simulink model "bh_SM_quad_and_PEND"  (R2019b)
settings: Solver=ode23t  StartTime=0.0  StopTime=200  FixedStep=0.001  RelTol=1e-5  EnableMultiTasking=on
values from neighbouring files (symbols this model uses):
  K = [0.0865712753524 0.00277244570809 -0.0192153083791 -0.00162453351485 3.32348361895e-08 -1.41900444311e-08 -0.0932413563659 2.38058592401e-06 6.56188614095e-09 -0.0932413743514 2.52459639721e-09 9.53911962763e-08 ... (84 elements, 4x21)]    [CONFIRMED_bh_CONT_DES_RESULTS.mat]    (also in CONFIRMED_bh_CONT_DES_RESULTS_DISCRETE.mat = [-4.44584196463e-19 1.60298866655e-18 6.22915677006e-18 0 -9; CONFIRMED_bh_CONT_DES_RESULTS_DISCRETE_PRE_19a_using_DARE_SOLVER.mat = [-0.000193022438438 0.000285510081841 0.000531074046333 0.00; CONFIRMED_bh_CONT_DES_RESULTS_DISCRETE_R2019b.mat = [3.0073494701e-20 1.31173839205e-18 -5.80308139081e-19 0 8.7; CONFIRMED_bh_CONT_DES_RESULTS_PRE_19a_using_CARE_SOLVER.mat = [3.8473936011e-07 5.10337913269e-05 5.50269068807e-05 0.0072)
  xme_dot_0 = (bRg .') * Vm_0(:)    [bh_func_for_lagr_mask_init.m]
undefined symbols (not defined in the file or in its folder): P_elec, P_mot, P_one_prop, P_pend, P_rot, P_veh, P_veh_no_props, sigbuilder_block, X, Y, Z
libraries: fl_lib x85, nesl_utility x39, sm_lib x30, simulink_extras x15, simulink x7, fl_ps_legacy_lib x7, bh_6dof_LIBRARY x1
(part 4 of 4)

== system bh_SM_quad_and_PEND/MODEL_SYS/bh_6DOF (Simscape)/Propellers/MOT_AERO_PROP_1/TQ_on_propeller/DC_mot_elec1 ==
  note: DC Motor - First Principle Equations
  note: L di/dt = V - R i - K_{emf}\fontsize{20}\omega
  PS Constant : fl_lib/Physical Signals/Sources/PS Constant  constant=L
      settings: AttributesFormatString=%<constant>
  PS Divide : fl_ps_legacy_lib/Legacy Physical Signals/Functions/PS Divide
      settings: SourceProductName=Simscape  SourceProductBaseCode=SS  InternalSimscapePortConfiguration="{\"Bottom\":[],\"Left\":[{\"id\":\"I1\",\"label\":\"\",\"type\":\"input\"},{\"id\":\"I2\",\"label\":\"\",\"type\":\"input\"}],\"Right\":[{\"id\":\"O\",\"label\":\"\",\"type\":\"output\"}],\"Top\":[]}"
  PS Gain1 : fl_ps_legacy_lib/Legacy Physical Signals/Functions/PS Gain  gain=Kb
      settings: AttributesFormatString=GAIN= %<gain>  SourceProductName=Simscape
  PS Gain2 : fl_ps_legacy_lib/Legacy Physical Signals/Functions/PS Gain  gain=R
      settings: AttributesFormatString=GAIN= %<gain>  SourceProductName=Simscape
  PS Gain3 : fl_ps_legacy_lib/Legacy Physical Signals/Functions/PS Gain  gain=K
      settings: AttributesFormatString=GAIN= %<gain>  SourceProductName=Simscape
  PS Integrator : fl_ps_legacy_lib/Legacy Physical Signals/Linear Operators/PS Integrator  x0=0
      settings: SourceProductName=Simscape  SourceProductBaseCode=SS  InternalSimscapePortConfiguration="{\"Bottom\":[],\"Left\":[{\"id\":\"I\",\"label\":\"\",\"type\":\"input\"}],\"Right\":[{\"id\":\"O\",\"label\":\"\",\"type\":\"output\"}],\"Top\":[]}"
  PS Subtract1 : fl_ps_legacy_lib/Legacy Physical Signals/Functions/PS Subtract
      settings: SourceProductName=Simscape  SourceProductBaseCode=SS
  PS Subtract2 : fl_ps_legacy_lib/Legacy Physical Signals/Functions/PS Subtract
      settings: SourceProductName=Simscape  SourceProductBaseCode=SS
  V : PMIOPort  Side=Left
  W : PMIOPort  Port=2  Side=Left
  Ki : PMIOPort  Port=3  Side=Right
  connections:
  PS Subtract1/LConn1 -- V/RConn1
  PS Gain1/RConn1 -- PS Subtract1/LConn2
  W/RConn1 -- PS Gain1/LConn1
  PS Subtract2/LConn1 -- PS Subtract1/RConn1
  PS Gain2/RConn1 -- PS Subtract2/LConn2
  PS Integrator/RConn1 -- PS Gain3/LConn1 -- PS Gain2/LConn1
  PS Divide/RConn1 -- PS Integrator/LConn1
  PS Subtract2/RConn1 -- PS Divide/LConn1
  PS Constant/RConn1 -- PS Divide/LConn2
  Ki/RConn1 -- PS Gain3/RConn1

== system bh_SM_quad_and_PEND/MODEL_SYS/bh_6DOF (Simscape)/Propellers/MOT_AERO_PROP_2/TQ_on_propeller/DC_mot_elec ==
  note: DC Motor - First Principle Equations
  note: L di/dt = V - R i - K_{emf}\fontsize{20}\omega
  PS Constant : fl_lib/Physical Signals/Sources/PS Constant  constant=L H
      settings: AttributesFormatString=|
      | %<constant>
      | UNITS = %<constant_unit>
  PS Divide : fl_lib/Physical Signals/Functions/PS Divide
      settings: SourceProductName=Simscape  SourceProductBaseCode=SS
  PS Gain1 : fl_lib/Physical Signals/Functions/PS Gain  gain=Kb V*s/rad
      settings: AttributesFormatString=|
      | GAIN= %<gain>
      | UNITS = %<gain_unit>
  PS Gain2 : fl_lib/Physical Signals/Functions/PS Gain  gain=R Ohm
      settings: AttributesFormatString=|
      | GAIN= %<gain>
      | UNITS = %<gain_unit>
  PS Gain3 : fl_lib/Physical Signals/Functions/PS Gain  gain=K N*m/A
      settings: AttributesFormatString=|
      | GAIN= %<gain>
      | UNITS = %<gain_unit>
  PS Integrator : fl_lib/Physical Signals/Linear Operators/PS Integrator  x0=0 A
      settings: AttributesFormatString=UNITS = %<x0_unit>  SourceProductName=Simscape  SourceProductBaseCode=SS
  PS Subtract1 : fl_lib/Physical Signals/Functions/PS Subtract
      settings: SourceProductName=Simscape
  PS Subtract2 : fl_lib/Physical Signals/Functions/PS Subtract
      settings: SourceProductName=Simscape
  V : PMIOPort  Side=Left
  W : PMIOPort  Port=2  Side=Left
  Ki : PMIOPort  Port=3  Side=Right
  connections:
  PS Subtract1/LConn1 -- V/RConn1
  PS Gain1/RConn1 -- PS Subtract1/LConn2
  W/RConn1 -- PS Gain1/LConn1
  PS Subtract2/LConn1 -- PS Subtract1/RConn1
  PS Gain2/RConn1 -- PS Subtract2/LConn2
  PS Integrator/RConn1 -- PS Gain3/LConn1 -- PS Gain2/LConn1
  PS Divide/RConn1 -- PS Integrator/LConn1
  PS Subtract2/RConn1 -- PS Divide/LConn1
  PS Constant/RConn1 -- PS Divide/LConn2
  Ki/RConn1 -- PS Gain3/RConn1

== system bh_SM_quad_and_PEND/MODEL_SYS/bh_6DOF (Simscape)/Propellers/MOT_AERO_PROP_2/TQ_on_propeller/DC_mot_elec1 ==
  note: DC Motor - First Principle Equations
  note: L di/dt = V - R i - K_{emf}\fontsize{20}\omega
  PS Constant : fl_lib/Physical Signals/Sources/PS Constant  constant=L
      settings: AttributesFormatString=%<constant>
  PS Divide : fl_lib/Physical Signals/Functions/PS Divide
      settings: SourceProductName=Simscape  SourceProductBaseCode=SS
  PS Gain1 : fl_lib/Physical Signals/Functions/PS Gain  gain=Kb
      settings: AttributesFormatString=GAIN= %<gain>
  PS Gain2 : fl_lib/Physical Signals/Functions/PS Gain  gain=R
      settings: AttributesFormatString=GAIN= %<gain>
  PS Gain3 : fl_lib/Physical Signals/Functions/PS Gain  gain=K
      settings: AttributesFormatString=GAIN= %<gain>
  PS Integrator : fl_lib/Physical Signals/Linear Operators/PS Integrator  x0=0 s
      settings: SourceProductName=Simscape  SourceProductBaseCode=SS
  PS Subtract1 : fl_lib/Physical Signals/Functions/PS Subtract
      settings: SourceProductName=Simscape
  PS Subtract2 : fl_lib/Physical Signals/Functions/PS Subtract
      settings: SourceProductName=Simscape
  V : PMIOPort  Side=Left
  W : PMIOPort  Port=2  Side=Left
  Ki : PMIOPort  Port=3  Side=Right
  connections:
  PS Subtract1/LConn1 -- V/RConn1
  PS Gain1/RConn1 -- PS Subtract1/LConn2
  W/RConn1 -- PS Gain1/LConn1
  PS Subtract2/LConn1 -- PS Subtract1/RConn1
  PS Gain2/RConn1 -- PS Subtract2/LConn2
  PS Integrator/RConn1 -- PS Gain3/LConn1 -- PS Gain2/LConn1
  PS Divide/RConn1 -- PS Integrator/LConn1
  PS Subtract2/RConn1 -- PS Divide/LConn1
  PS Constant/RConn1 -- PS Divide/LConn2
  Ki/RConn1 -- PS Gain3/RConn1

== system bh_SM_quad_and_PEND/MODEL_SYS/bh_6DOF (Simscape)/Propellers/MOT_AERO_PROP_3/TQ_on_propeller/DC_mot_elec ==
  note: DC Motor - First Principle Equations
  note: L di/dt = V - R i - K_{emf}\fontsize{20}\omega
  PS Constant : fl_lib/Physical Signals/Sources/PS Constant  constant=L H
      settings: AttributesFormatString=|
      | %<constant>
      | UNITS = %<constant_unit>
  PS Divide : fl_lib/Physical Signals/Functions/PS Divide
      settings: SourceProductName=Simscape  SourceProductBaseCode=SS
  PS Gain1 : fl_lib/Physical Signals/Functions/PS Gain  gain=Kb V*s/rad
      settings: AttributesFormatString=|
      | GAIN= %<gain>
      | UNITS = %<gain_unit>
  PS Gain2 : fl_lib/Physical Signals/Functions/PS Gain  gain=R Ohm
      settings: AttributesFormatString=|
      | GAIN= %<gain>
      | UNITS = %<gain_unit>
  PS Gain3 : fl_lib/Physical Signals/Functions/PS Gain  gain=K N*m/A
      settings: AttributesFormatString=|
      | GAIN= %<gain>
      | UNITS = %<gain_unit>
  PS Integrator : fl_lib/Physical Signals/Linear Operators/PS Integrator  x0=0 A
      settings: AttributesFormatString=UNITS = %<x0_unit>  SourceProductName=Simscape  SourceProductBaseCode=SS
  PS Subtract1 : fl_lib/Physical Signals/Functions/PS Subtract
      settings: SourceProductName=Simscape
  PS Subtract2 : fl_lib/Physical Signals/Functions/PS Subtract
      settings: SourceProductName=Simscape
  V : PMIOPort  Side=Left
  W : PMIOPort  Port=2  Side=Left
  Ki : PMIOPort  Port=3  Side=Right
  connections:
  PS Subtract1/LConn1 -- V/RConn1
  PS Gain1/RConn1 -- PS Subtract1/LConn2
  W/RConn1 -- PS Gain1/LConn1
  PS Subtract2/LConn1 -- PS Subtract1/RConn1
  PS Gain2/RConn1 -- PS Subtract2/LConn2
  PS Integrator/RConn1 -- PS Gain3/LConn1 -- PS Gain2/LConn1
  PS Divide/RConn1 -- PS Integrator/LConn1
  PS Subtract2/RConn1 -- PS Divide/LConn1
  PS Constant/RConn1 -- PS Divide/LConn2
  Ki/RConn1 -- PS Gain3/RConn1

== system bh_SM_quad_and_PEND/MODEL_SYS/bh_6DOF (Simscape)/Propellers/MOT_AERO_PROP_3/TQ_on_propeller/DC_mot_elec1 ==
  note: DC Motor - First Principle Equations
  note: L di/dt = V - R i - K_{emf}\fontsize{20}\omega
  PS Constant : fl_lib/Physical Signals/Sources/PS Constant  constant=L
      settings: AttributesFormatString=%<constant>
  PS Divide : fl_lib/Physical Signals/Functions/PS Divide
      settings: SourceProductName=Simscape  SourceProductBaseCode=SS
  PS Gain1 : fl_lib/Physical Signals/Functions/PS Gain  gain=Kb
      settings: AttributesFormatString=GAIN= %<gain>
  PS Gain2 : fl_lib/Physical Signals/Functions/PS Gain  gain=R
      settings: AttributesFormatString=GAIN= %<gain>
  PS Gain3 : fl_lib/Physical Signals/Functions/PS Gain  gain=K
      settings: AttributesFormatString=GAIN= %<gain>
  PS Integrator : fl_lib/Physical Signals/Linear Operators/PS Integrator  x0=0 s
      settings: SourceProductName=Simscape  SourceProductBaseCode=SS
  PS Subtract1 : fl_lib/Physical Signals/Functions/PS Subtract
      settings: SourceProductName=Simscape
  PS Subtract2 : fl_lib/Physical Signals/Functions/PS Subtract
      settings: SourceProductName=Simscape
  V : PMIOPort  Side=Left
  W : PMIOPort  Port=2  Side=Left
  Ki : PMIOPort  Port=3  Side=Right
  connections:
  PS Subtract1/LConn1 -- V/RConn1
  PS Gain1/RConn1 -- PS Subtract1/LConn2
  W/RConn1 -- PS Gain1/LConn1
  PS Subtract2/LConn1 -- PS Subtract1/RConn1
  PS Gain2/RConn1 -- PS Subtract2/LConn2
  PS Integrator/RConn1 -- PS Gain3/LConn1 -- PS Gain2/LConn1
  PS Divide/RConn1 -- PS Integrator/LConn1
  PS Subtract2/RConn1 -- PS Divide/LConn1
  PS Constant/RConn1 -- PS Divide/LConn2
  Ki/RConn1 -- PS Gain3/RConn1

== system bh_SM_quad_and_PEND/MODEL_SYS/bh_6DOF (Simscape)/Propellers/MOT_AERO_PROP_4/TQ_on_propeller/DC_mot_elec ==
  note: DC Motor - First Principle Equations
  note: L di/dt = V - R i - K_{emf}\fontsize{20}\omega
  PS Constant : fl_lib/Physical Signals/Sources/PS Constant  constant=L H
      settings: AttributesFormatString=|
      | %<constant>
      | UNITS = %<constant_unit>
  PS Divide : fl_lib/Physical Signals/Functions/PS Divide
      settings: SourceProductName=Simscape  SourceProductBaseCode=SS
  PS Gain1 : fl_lib/Physical Signals/Functions/PS Gain  gain=Kb V*s/rad
      settings: AttributesFormatString=|
      | GAIN= %<gain>
      | UNITS = %<gain_unit>
  PS Gain2 : fl_lib/Physical Signals/Functions/PS Gain  gain=R Ohm
      settings: AttributesFormatString=|
      | GAIN= %<gain>
      | UNITS = %<gain_unit>
  PS Gain3 : fl_lib/Physical Signals/Functions/PS Gain  gain=K N*m/A
      settings: AttributesFormatString=|
      | GAIN= %<gain>
      | UNITS = %<gain_unit>
  PS Integrator : fl_lib/Physical Signals/Linear Operators/PS Integrator  x0=0 A
      settings: AttributesFormatString=UNITS = %<x0_unit>  SourceProductName=Simscape  SourceProductBaseCode=SS
  PS Subtract1 : fl_lib/Physical Signals/Functions/PS Subtract
      settings: SourceProductName=Simscape
  PS Subtract2 : fl_lib/Physical Signals/Functions/PS Subtract
      settings: SourceProductName=Simscape
  V : PMIOPort  Side=Left
  W : PMIOPort  Port=2  Side=Left
  Ki : PMIOPort  Port=3  Side=Right
  connections:
  PS Subtract1/LConn1 -- V/RConn1
  PS Gain1/RConn1 -- PS Subtract1/LConn2
  W/RConn1 -- PS Gain1/LConn1
  PS Subtract2/LConn1 -- PS Subtract1/RConn1
  PS Gain2/RConn1 -- PS Subtract2/LConn2
  PS Integrator/RConn1 -- PS Gain3/LConn1 -- PS Gain2/LConn1
  PS Divide/RConn1 -- PS Integrator/LConn1
  PS Subtract2/RConn1 -- PS Divide/LConn1
  PS Constant/RConn1 -- PS Divide/LConn2
  Ki/RConn1 -- PS Gain3/RConn1

== system bh_SM_quad_and_PEND/MODEL_SYS/bh_6DOF (Simscape)/Propellers/MOT_AERO_PROP_4/TQ_on_propeller/DC_mot_elec1 ==
  note: DC Motor - First Principle Equations
  note: L di/dt = V - R i - K_{emf}\fontsize{20}\omega
  PS Constant : fl_lib/Physical Signals/Sources/PS Constant  constant=L
      settings: AttributesFormatString=%<constant>
  PS Divide : fl_lib/Physical Signals/Functions/PS Divide
      settings: SourceProductName=Simscape  SourceProductBaseCode=SS
  PS Gain1 : fl_lib/Physical Signals/Functions/PS Gain  gain=Kb
      settings: AttributesFormatString=GAIN= %<gain>
  PS Gain2 : fl_lib/Physical Signals/Functions/PS Gain  gain=R
      settings: AttributesFormatString=GAIN= %<gain>
  PS Gain3 : fl_lib/Physical Signals/Functions/PS Gain  gain=K
      settings: AttributesFormatString=GAIN= %<gain>
  PS Integrator : fl_lib/Physical Signals/Linear Operators/PS Integrator  x0=0 s
      settings: SourceProductName=Simscape  SourceProductBaseCode=SS
  PS Subtract1 : fl_lib/Physical Signals/Functions/PS Subtract
      settings: SourceProductName=Simscape
  PS Subtract2 : fl_lib/Physical Signals/Functions/PS Subtract
      settings: SourceProductName=Simscape
  V : PMIOPort  Side=Left
  W : PMIOPort  Port=2  Side=Left
  Ki : PMIOPort  Port=3  Side=Right
  connections:
  PS Subtract1/LConn1 -- V/RConn1
  PS Gain1/RConn1 -- PS Subtract1/LConn2
  W/RConn1 -- PS Gain1/LConn1
  PS Subtract2/LConn1 -- PS Subtract1/RConn1
  PS Gain2/RConn1 -- PS Subtract2/LConn2
  PS Integrator/RConn1 -- PS Gain3/LConn1 -- PS Gain2/LConn1
  PS Divide/RConn1 -- PS Integrator/LConn1
  PS Subtract2/RConn1 -- PS Divide/LConn1
  PS Constant/RConn1 -- PS Divide/LConn2
  Ki/RConn1 -- PS Gain3/RConn1

== matlab function bh_SM_quad_and_PEND/CONT_SYS W_MOT_CMDS2/FM_to_w2 ==
  data: L input; w2_cmd output; Thrust_const input; Twist_const input; Thrust input; TQ_roll_X input; TQ_pit_Y input; TQ_yaw_Z input
function w2_cmd = FMtow2(L, Thrust_const, Twist_const, Thrust, TQ_roll_X, TQ_pit_Y, TQ_yaw_Z)
%#codegen

    % simplify the variable names
    b = Thrust_const;
    k = Twist_const;

    % construct the co-efficient matrix:
    %  F_and_M = C * w^2
    %
    C = [     b,    b,    b,    b;
              0,    b*L,  0,   -b*L;
             -b*L,  0,    b*L,  0;
             -k,    k,   -k,    k; ];

    % used Symbolic toolbox to compute inv(C)
    C_inv = [
             1/(4*b),          0, -1/(2*L*b), -1/(4*k);
             1/(4*b),  1/(2*L*b),          0,  1/(4*k);
             1/(4*b),          0,  1/(2*L*b), -1/(4*k);
             1/(4*b), -1/(2*L*b),          0,  1/(4*k);
            ];
    % solve for the w^2 vec
    F_and_M_col = [Thrust, TQ_roll_X, TQ_pit_Y, TQ_yaw_Z].' ;
    w2_cmd      = C_inv * F_and_M_col; 
    % check that ALL w^2 >=0
    tf_col      = (w2_cmd >= 0);
%     if( ~all(tf_col) )
%         w2_cmd = lsqnonneg(C, F_and_M_col);
%     end
%     
%     tf_again_col = (w2_cmd >= 0);
%     assert(all(tf_again_col), 'ERROR: ohh dear some w2 are NEGATIVE !')
   
%     for kk=1:4
%       fprintf('\n ... [%.16f]', w2_cmd(kk) );
%     end
%     fprintf('\n -----------------------------------------------');
    assert(all(tf_col), 'ERROR: ohh dear some w2 are NEGATIVE !')
    
% 
%      if( ~all(tf_col) )
%        fprintf('\n ..... WHAT HAPPENED !');
%      end
%     assert(all(tf_col), 'ERROR: ohh dear some w2 are NEGATIVE !')
   %assert(false, 'ERROR: some w2 are NEGATIVE !')
end

== matlab function bh_SM_quad_and_PEND/a_circle1/MATLAB Function ==
  data: t_clock input; XYZ output; t_to_start input; RADIUS input; ztgt input; w input
function XYZ = fcn(t_clock, t_to_start, RADIUS, ztgt, w)

t    = t_clock - t_to_start;

theta = w*t;

x = RADIUS * cos(theta);
y = RADIUS * sin(theta);
z = ztgt;


XYZ = [x;y;z];

== matlab function bh_SM_quad_and_PEND/MODEL_SYS/bh_6DOF (Simscape)/6DOF_JOINT_SYS/Angular_MEAS/Calc Euler_rates/my_euler_rates ==
  data: theta input; euler_rates output; psi input; p input; q input; r input
function euler_rates = my_euler_rates(theta,psi,p,q,r)
%#codegen

%    This function was generated by the Symbolic Math Toolbox version 7.0.
%    09-Jun-2016 10:28:25

euler_rates = [(r.*cos(psi)+q.*sin(psi))./cos(theta);
                q.*cos(psi)-r.*sin(psi);
               (p.*cos(theta)+r.*cos(psi).*sin(theta)+q.*sin(psi).*sin(theta))./cos(theta)];

== matlab function bh_SM_quad_and_PEND/MODEL_SYS/bh_6DOF (Simscape)/6DOF_JOINT_SYS/Angular_MEAS/calc_DCM ==
  data: bRg input; eul_vec output
function eul_vec = calc_eul_ang(bRg)
%#codegen

% bRg = [ ...
%                               cos(phi)*cos(theta),                              cos(theta)*sin(phi),         -sin(theta);
%  cos(phi)*sin(psi)*sin(theta) - cos(psi)*sin(phi), cos(phi)*cos(psi) + sin(phi)*sin(psi)*sin(theta), cos(theta)*sin(psi);
%  sin(phi)*sin(psi) + cos(phi)*cos(psi)*sin(theta), cos(psi)*sin(phi)*sin(theta) - cos(phi)*sin(psi), cos(psi)*cos(theta);
%  ];

%phi, theta, psi


theta = asin( -bRg(1,3)  ); %  theta is in the range [-pi/2, pi/2]

% Recall the DOC on atan2()
%     atan2(Y,X) is the four quadrant arctangent of the elements of X and Y
%     such that -pi <= atan2(Y,X) <= pi

Y   = bRg(1,2);
X   = bRg(1,1);
phi = atan2(Y,X);

Y   = bRg(2,3);
X   = bRg(3,3);
psi = atan2(Y,X);

% now populate the output
eul_vec    = zeros(3,1);

eul_vec(1) = phi;
eul_vec(2) = theta;
eul_vec(3) = psi;

end

== matlab function bh_SM_quad_and_PEND/MODEL_SYS/bh_6DOF (Simscape)/PEND_SYS/Pend_Angular_MEAS/Calc Euler_rates/my_euler_rates ==
  data: theta input; euler_rates output; psi input; p input; q input; r input
function euler_rates = my_euler_rates(theta,psi,p,q,r)
%#codegen

%    This function was generated by the Symbolic Math Toolbox version 7.0.
%    09-Jun-2016 10:28:25

euler_rates = [(r.*cos(psi)+q.*sin(psi))./cos(theta);
                q.*cos(psi)-r.*sin(psi);
               (p.*cos(theta)+r.*cos(psi).*sin(theta)+q.*sin(psi).*sin(theta))./cos(theta)];

== matlab function bh_SM_quad_and_PEND/MODEL_SYS/bh_6DOF (Simscape)/PEND_SYS/Pend_Angular_MEAS/calc_DCM ==
  data: bRg input; eul_vec output
function eul_vec = calc_eul_ang(bRg)
%#codegen

% bRg = [ ...
%                               cos(phi)*cos(theta),                              cos(theta)*sin(phi),         -sin(theta);
%  cos(phi)*sin(psi)*sin(theta) - cos(psi)*sin(phi), cos(phi)*cos(psi) + sin(phi)*sin(psi)*sin(theta), cos(theta)*sin(psi);
%  sin(phi)*sin(psi) + cos(phi)*cos(psi)*sin(theta), cos(psi)*sin(phi)*sin(theta) - cos(phi)*sin(psi), cos(psi)*cos(theta);
%  ];

%phi, theta, psi


theta = asin( -bRg(1,3)  ); %  theta is in the range [-pi/2, pi/2]

% Recall the DOC on atan2()
%     atan2(Y,X) is the four quadrant arctangent of the elements of X and Y
%     such that -pi <= atan2(Y,X) <= pi

Y   = bRg(1,2);
X   = bRg(1,1);
phi = atan2(Y,X);

Y   = bRg(2,3);
X   = bRg(3,3);
psi = atan2(Y,X);

% now populate the output
eul_vec    = zeros(3,1);

eul_vec(1) = phi;
eul_vec(2) = theta;
eul_vec(3) = psi;

end

== matlab function bh_SM_quad_and_PEND/CONT_SYS W_MOT_CMDS2/w2toFM1 ==
  data: L input; Tbz_col output; Thrust_const input; Twist_const input; w2_col input; Mbz_col output; wM_col output
function [Tbz_col, Mbz_col, wM_col] = w2toFM(L, Thrust_const, Twist_const, w2_col)
%#codegen

    % simplify the variable names
    b = Thrust_const;
    k = Twist_const;

    % construct the co-efficient matrix:
    %  F_and_M = C * w^2
    
%     C = [     b,    b,    b,    b;
%               0,    b*L,  0,   -b*L;
%              -b*L,  0,    b*L,  0;
%              -k,    k,   -k,    k; ];

    Tbz_col = [ b; b; b; b ]  .*  w2_col;     
    Mbz_col = [-k; k;-k; k ]  .*  w2_col;          
    wM_col  = [ 1;-1; 1;-1 ]  .*  sqrt(w2_col); 
end
